simulink model "fypimc01"  (R2021a)
settings: Solver=VariableStepAuto  StartTime=0.0  StopTime=100.0  RelTol=1e-3
settings Model: Creator=mluser  LastModifiedBy=mluser

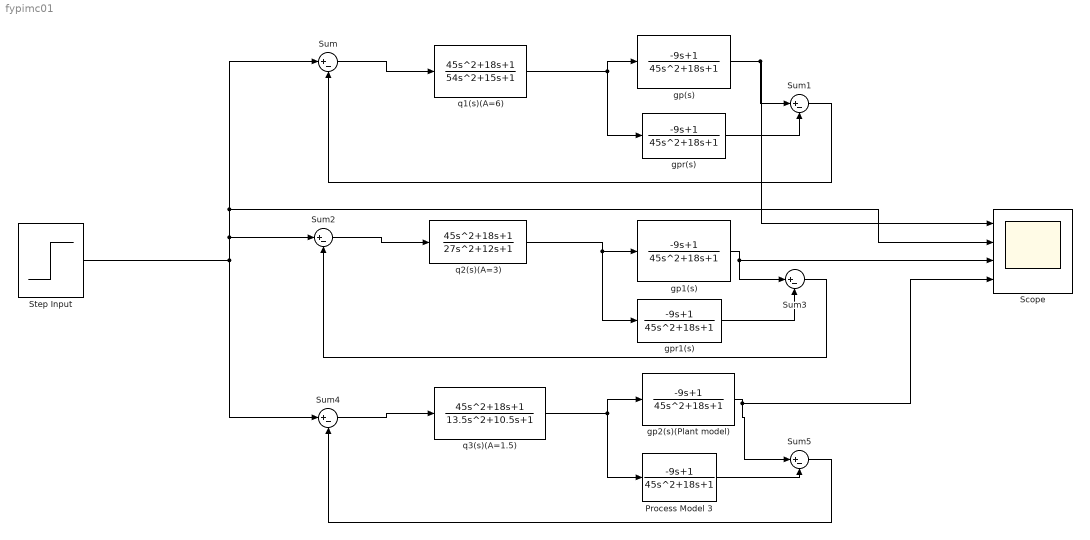
== system fypimc01 ==
  Process Model 3 : TransferFcn  Numerator=[-9 1]  Denominator=[45 18 1]
  Scope : Scope  NumInputPorts=4
  Step Input : Step  SampleTime=0
  Sum{,1..5} (6 alike) : Sum  Inputs=|+-
  gp(s) : TransferFcn  Numerator=[-9 1]  Denominator=[45 18 1]  ContinuousStateAttributes='gp(s)(Plant model)'
  gp1(s) : TransferFcn  Numerator=[-9 1]  Denominator=[45 18 1]
  gp2(s)(Plant model) : TransferFcn  Numerator=[-9 1]  Denominator=[45 18 1]
  gpr(s) : TransferFcn  Numerator=[-9 1]  Denominator=[45 18 1]
  gpr1(s) : TransferFcn  Numerator=[-9 1]  Denominator=[45 18 1]
  q1(s)(A=6) : TransferFcn  Numerator=[45 18 1]  Denominator=[54 15 1]  ParameterTunability=Unconstrained  ContinuousStateAttributes='q1(s)(A=6)'
  q2(s)(A=3) : TransferFcn  Numerator=[45 18 1]  Denominator=[27 12 1]  ParameterTunability=Optimized
  q3(s)(A=1.5) : TransferFcn  Numerator=[45 18 1]  Denominator=[13.5 10.5 1]  ParameterTunability=Optimized
  wires:
  Sum/1 -> q1(s)(A=6)/1
  q1(s)(A=6)/1 -> gp(s)/1, gpr(s)/1
  gp(s)/1 -> Sum1/1, Scope/1
  gpr(s)/1 -> Sum1/2
  Sum1/1 -> Sum/2
  q2(s)(A=3)/1 -> gp1(s)/1, gpr1(s)/1
  gp1(s)/1 -> Sum3/1, Scope/3
  gpr1(s)/1 -> Sum3/2
  Sum2/1 -> q2(s)(A=3)/1
  Sum3/1 -> Sum2/2
  q3(s)(A=1.5)/1 -> Process Model 3/1, gp2(s)(Plant model)/1
  Step Input/1 -> Sum/1, Scope/2, Sum2/1, Sum4/1
  gp2(s)(Plant model)/1 -> Sum5/1, Scope/4
  Process Model 3/1 -> Sum5/2
  Sum4/1 -> q3(s)(A=1.5)/1
  Sum5/1 -> Sum4/2
